simulink model "PruebaZ"  (R2018b)
settings: Solver=VariableStepAuto  StartTime=0.0  StopTime=ttotal  RelTol=1e-3
values from neighbouring files (symbols this model uses):
  tmuestra = 0.05    [ABCIncremental.m]    (also in ABCLQR.m)
  Yr = 0.05    [ABCIncremental.m]    (also in ABCLQR.m = 0.1)
undefined symbols (not defined in the file or in its folder): A1, A2, A3, B1, B2, B3, C1, C2, C3, ControlDiscretoBAB
settings Model: Creator=pablo  LastModifiedBy=pablo

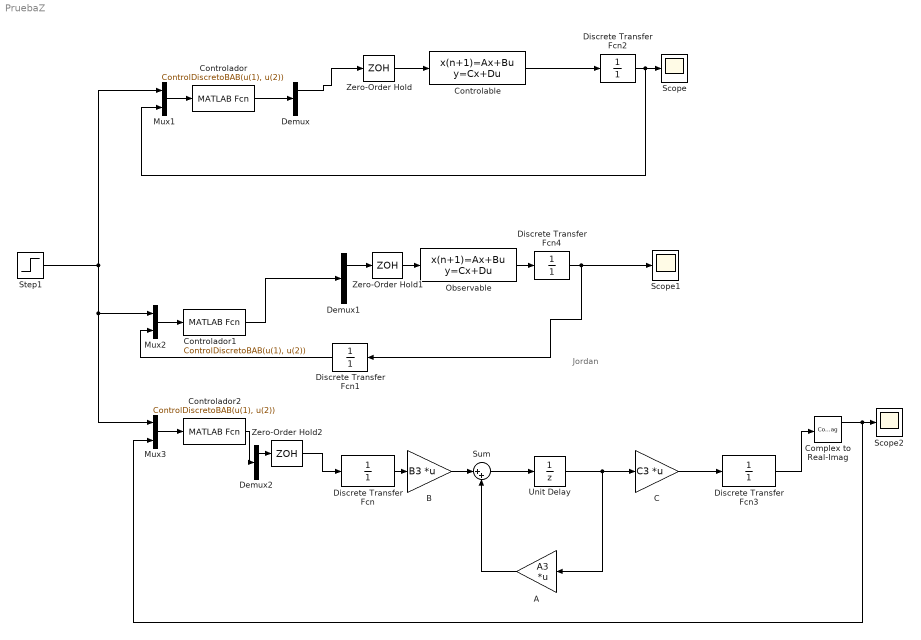
== system PruebaZ ==
  note: Jordan
  A : Gain  Gain=A3  Multiplication=Matrix(K*u)
  B : Gain  Gain=B3  Multiplication=Matrix(K*u)
  C : Gain  Gain=C3  Multiplication=Matrix(K*u)
  Complex to Real-Imag : ComplexToRealImag
  Controlable : DiscreteStateSpace  A=A1  B=B1  C=C1  D=0  SampleTime=tmuestra
  Controlador : MATLABFcn  MATLABFcn=ControlDiscretoBAB(u(1), u(2))  OutputDimensions=2
  Controlador1 : MATLABFcn  MATLABFcn=ControlDiscretoBAB(u(1), u(2))  OutputDimensions=2
  Controlador2 : MATLABFcn  MATLABFcn=ControlDiscretoBAB(u(1), u(2))  OutputDimensions=2
  Demux : Demux  Outputs=2
  Demux1 : Demux  Outputs=2
  Demux2 : Demux  Outputs=2
  Discrete Transfer Fcn{,1..4} (5 alike) : DiscreteTransferFcn  Denominator=[1]  SampleTime=tmuestra
  Mux1 : Mux  Inputs=2
  Mux2 : Mux  Inputs=2
  Mux3 : Mux  Inputs=2
  Observable : DiscreteStateSpace  A=A2  B=B2  C=C2  D=0  SampleTime=tmuestra
  Scope : Scope
  Scope1 : Scope
  Scope2 : Scope
  Step1 : Step  After=Yr  SampleTime=tmuestra
  Sum : Sum  Inputs=|++
  Unit Delay : UnitDelay  SampleTime=tmuestra
  Zero-Order Hold : ZeroOrderHold  SampleTime=tmuestra
  Zero-Order Hold1 : ZeroOrderHold  SampleTime=tmuestra
  Zero-Order Hold2 : ZeroOrderHold  SampleTime=tmuestra
  wires:
  Observable/1 -> Discrete Transfer Fcn4/1
  A/1 -> Sum/2
  B/1 -> Sum/1
  Sum/1 -> Unit Delay/1
  Unit Delay/1 -> C/1, A/1
  Discrete Transfer Fcn/1 -> B/1
  C/1 -> Discrete Transfer Fcn3/1
  Mux1/1 -> Controlador/1
  Mux2/1 -> Controlador1/1
  Mux3/1 -> Controlador2/1
  Step1/1 -> Mux3/1, Mux2/1, Mux1/1
  Controlador1/1 -> Demux1/1
  Controlador/1 -> Demux/1
  Demux1/1 -> Zero-Order Hold1/1
  Controlador2/1 -> Demux2/1
  Discrete Transfer Fcn1/1 -> Mux2/2
  Controlable/1 -> Discrete Transfer Fcn2/1
  Complex to Real-Imag/1 -> Mux3/2, Scope2/1
  Zero-Order Hold/1 -> Controlable/1
  Demux/1 -> Zero-Order Hold/1
  Zero-Order Hold1/1 -> Observable/1
  Zero-Order Hold2/1 -> Discrete Transfer Fcn/1
  Demux2/1 -> Zero-Order Hold2/1
  Discrete Transfer Fcn2/1 -> Mux1/2, Scope/1
  Discrete Transfer Fcn4/1 -> Scope1/1, Discrete Transfer Fcn1/1
  Discrete Transfer Fcn3/1 -> Complex to Real-Imag/1
